simulink model "HydraulicSimulink"  (R2017a)
settings: Solver=ode23  StartTime=0.0  StopTime=10.0  RelTol=1e-3
values from neighbouring files (symbols this model uses):
  A = (A1 + A2) / 2    (= 0.00180641577581)    [ex6Parameter.m]
  a = [-df/M, A/M, -A/M ... (first row only)    [ex6Parameter.m]
  A2 = A1 - pi*1e-4    (= 0.00164933614313)    [ex6Parameter.m]
  b = [-1/M; 0; 0]    [ex6Parameter.m]
  c = [1,0,0 ... (first row only)    [ex6Parameter.m]
  Cf = V / Bulk    (= 6.32245521535e-13)    [ex6Parameter.m]
  d = [0;0;0]    [ex6Parameter.m]
  df = 200    [ex6Parameter.m]
  M = 100    [ex6Parameter.m]
  P1eq = Ps - (A*Veq/Rv/Xv)^2    [ex6Parameter.m]
  P2eq = (A*Veq/Rv/Xv)^2    [ex6Parameter.m]
  Ps = 20e6    (= 20000000)    [ex6Parameter.m]
  Rv = 1e-4    (= 0.0001)    [ex6Parameter.m]
  Veq = select(Veq1, Veq2)    [ex6Parameter.m]
  Xv = 1e-2    (= 0.01)    [ex6Parameter.m]
settings Model: Creator=99641  LastModifiedBy=99641

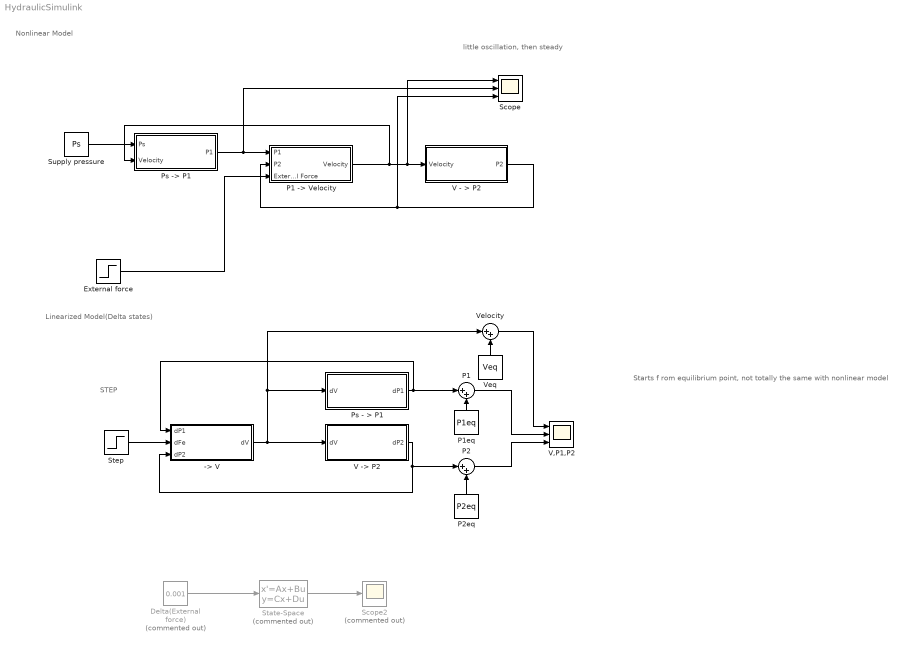
== system HydraulicSimulink ==
  note: STEP
  note: Starts f rom equilibrium point, not totally the same with nonlinear model
  note: Linearized Model(Delta states)
  note: Nonlinear Model
  note: little oscillation, then steady
  -> V : Subsystem
  Delta(External force) : Constant  Commented=on  Value=0.001
  External force : Step  After=0  SampleTime=0
  P1 : Sum  Inputs=|++
  "P1 -> Velocity" : Subsystem
  P1eq : Constant  Value=P1eq
  P2 : Sum  Inputs=|++  LockScale=on
  P2eq : Constant  Value=P2eq
  "Ps - > P1 " : Subsystem
  "Ps -> P1" : Subsystem
  Scope : Scope  NumInputPorts=3
  Scope2 : Scope  Commented=on
  State-Space : StateSpace  Commented=on  A=a  B=b  C=c  D=d  X0=0  ContinuousStateAttributes='Velocity.P1.P2'
  Step : Step  After=0.01  SampleTime=0
  Supply pressure : Constant  Value=Ps
  V - > P2 : Subsystem
  "V -> P2" : Subsystem
  "V,P1,P2 " : Scope  NumInputPorts=3
  Velocity : Sum  Inputs=|++
  Veq : Constant  Value=Veq
  wires:
  V - > P2/1(P2) -> Scope/3, "P1 -> Velocity"/2(P2)
  Supply pressure/1 -> "Ps -> P1"/1("Ps ")
  "Ps -> P1"/1(P1) -> Scope/2, "P1 -> Velocity"/1(P1)
  "P1 -> Velocity"/1(Velocity) -> "Ps -> P1"/2(Velocity), Scope/1, V - > P2/1(Velocity)
  External force/1 -> "P1 -> Velocity"/3(External Force)
  "Ps - > P1 "/1("dP1 ") -> P1/1, -> V/1(dP1)
  -> V/1("dV ") -> Velocity/1, "Ps - > P1 "/1(dV), "V -> P2"/1(dV)
  State-Space/1 -> Scope2/1
  Delta(External force)/1 -> State-Space/1
  P1/1 -> "V,P1,P2 "/2
  P1eq/1 -> P1/2
  Veq/1 -> Velocity/2
  Velocity/1 -> "V,P1,P2 "/1
  P2eq/1 -> P2/2
  "V -> P2"/1("dP2 ") -> P2/1, -> V/3(dP2)
  P2/1 -> "V,P1,P2 "/3
  Step/1 -> -> V/2(dFe)

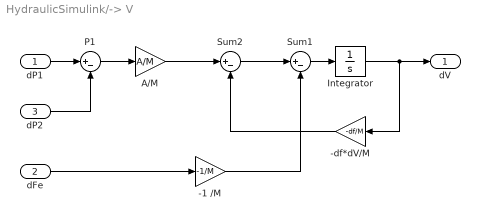
== system HydraulicSimulink/-> V ==
  dP1 : Inport
  dFe : Inport  Port=2
  dP2 : Inport  Port=3
  -1 /M : Gain  Gain=-1/M
  -df*dV/M : Gain  Gain=-df/M
  A/M : Gain  Gain=A/M
  Integrator : Integrator
  P1 : Sum  Inputs=|+-
  Sum1 : Sum  Inputs=|+-
  Sum2 : Sum  Inputs=|+-
  "dV " : Outport
  wires:
  -1 /M/1 -> Sum1/2
  dFe/1 -> -1 /M/1
  Sum1/1 -> Integrator/1
  Integrator/1 -> -df*dV/M/1, "dV "/1
  P1/1 -> A/M/1
  dP1/1 -> P1/1
  dP2/1 -> P1/2
  Sum2/1 -> Sum1/1
  A/M/1 -> Sum2/1
  -df*dV/M/1 -> Sum2/2

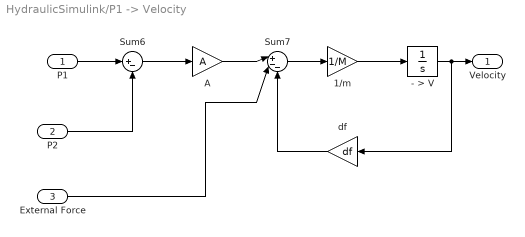
== system HydraulicSimulink/P1 -> Velocity ==
  P1 : Inport
  P2 : Inport  Port=2
  External Force : Inport  Port=3
  - > V : Integrator
  1/m : Gain  Gain=1/M
  A : Gain  Gain=A
  Sum6 : Sum  Inputs=|+-
  Sum7 : Sum  Inputs=|+--
  df : Gain  Gain=df
  Velocity : Outport
  wires:
  Sum6/1 -> A/1
  1/m/1 -> - > V/1
  Sum7/1 -> 1/m/1
  df/1 -> Sum7/3
  A/1 -> Sum7/1
  - > V/1 -> df/1, Velocity/1
  P1/1 -> Sum6/1
  P2/1 -> Sum6/2
  External Force/1 -> Sum7/2

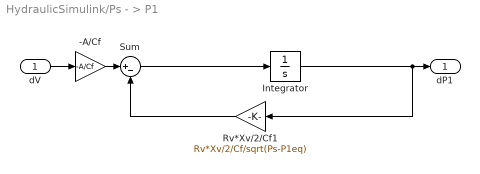
== system HydraulicSimulink/Ps - > P1  ==
  dV : Inport
  -A/Cf : Gain  Gain=-A/Cf
  Integrator : Integrator
  Rv*Xv/2/Cf1 : Gain  Gain=Rv*Xv/2/Cf/sqrt(Ps-P1eq)
  Sum : Sum  Inputs=|+-
  "dP1 " : Outport
  wires:
  Integrator/1 -> Rv*Xv/2/Cf1/1, "dP1 "/1
  Sum/1 -> Integrator/1
  Rv*Xv/2/Cf1/1 -> Sum/2
  dV/1 -> -A/Cf/1
  -A/Cf/1 -> Sum/1

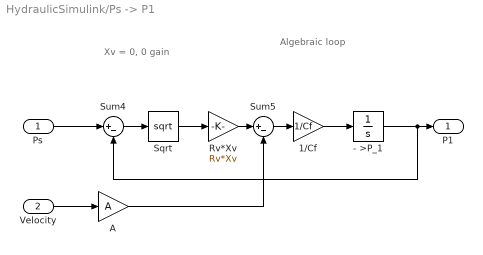
== system HydraulicSimulink/Ps -> P1 ==
  note: Algebraic loop
  note: Xv = 0, 0 gain
  "Ps " : Inport
  Velocity : Inport  Port=2
  "- >P_1 " : Integrator
  1/Cf : Gain  Gain=1/Cf
  A : Gain  Gain=A
  Rv*Xv : Gain  Gain=Rv*Xv
  Sqrt : Sqrt  SaturateOnIntegerOverflow=on
  Sum4 : Sum  Inputs=|+-
  Sum5 : Sum  Inputs=|+-
  P1 : Outport
  wires:
  "Ps "/1 -> Sum4/1
  Rv*Xv/1 -> Sum5/1
  1/Cf/1 -> "- >P_1 "/1
  Sum5/1 -> 1/Cf/1
  "- >P_1 "/1 -> Sum4/2, P1/1
  Velocity/1 -> A/1
  A/1 -> Sum5/2
  Sum4/1 -> Sqrt/1
  Sqrt/1 -> Rv*Xv/1

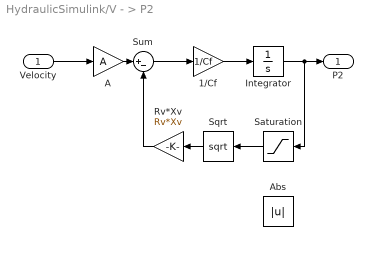
== system HydraulicSimulink/V - > P2 ==
  Velocity : Inport
  1/Cf : Gain  Gain=1/Cf
  A : Gain  Gain=A
  Abs : Abs
  Integrator : Integrator
  Rv*Xv : Gain  Gain=Rv*Xv
  Saturation : Saturate  UpperLimit=Ps  LowerLimit=0  ZeroCross=off
  Sqrt : Sqrt  SaturateOnIntegerOverflow=on
  Sum : Sum  Inputs=|+-
  P2 : Outport
  wires:
  Velocity/1 -> A/1
  Sum/1 -> 1/Cf/1
  A/1 -> Sum/1
  1/Cf/1 -> Integrator/1
  Sqrt/1 -> Rv*Xv/1
  Rv*Xv/1 -> Sum/2
  Saturation/1 -> Sqrt/1
  Integrator/1 -> Saturation/1, P2/1

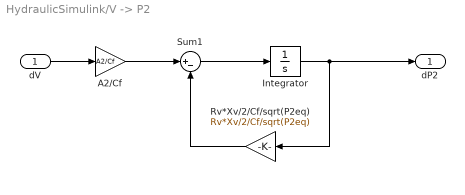
== system HydraulicSimulink/V -> P2 ==
  dV : Inport
  A2/Cf : Gain  Gain=A2/Cf
  Integrator : Integrator
  Rv*Xv/2/Cf/sqrt(P2eq) : Gain  Gain=Rv*Xv/2/Cf/sqrt(P2eq)
  Sum1 : Sum  Inputs=|+-
  "dP2 " : Outport
  wires:
  Sum1/1 -> Integrator/1
  dV/1 -> A2/Cf/1
  A2/Cf/1 -> Sum1/1
  Integrator/1 -> Rv*Xv/2/Cf/sqrt(P2eq)/1, "dP2 "/1
  Rv*Xv/2/Cf/sqrt(P2eq)/1 -> Sum1/2
